simulink model "NL_RE"  (R2015a)
settings: Solver=ode4  StartTime=0.0  StopTime=10.0  RelTol=1e-3
values from neighbouring files (symbols this model uses):
  K = [0 K(2)]    [CommandeEE2.m]
undefined symbols (not defined in the file or in its folder): Cn, EE2, EE2_bf, J2, Kc, Ke, Kg, Kr, Ks, L, mu, obsver, R, Rchn, rCn, rRch
settings Model: Creator=sylvain  LastModifiedBy=Lucien
settings OptimizationCC: ExpressionDepthLimit=2147483647
settings DebuggingCC: UnderspecifiedInitializationDetection=Classic  MergeDetectMultiDrivingBlocksExec=none  SolverPrmCheckMsg=warning  StateNameClashWarn=warning

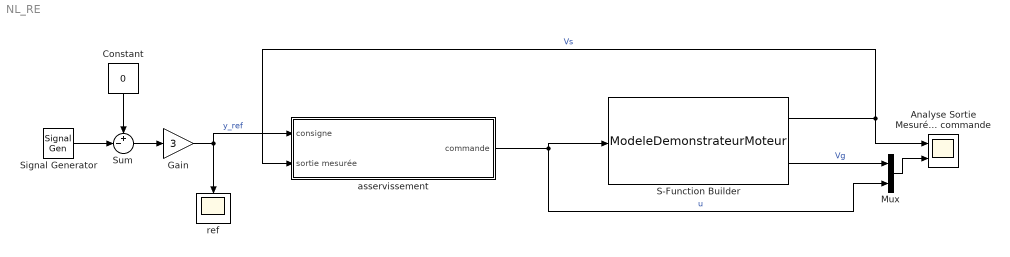
== system NL_RE ==
  Analyse Sortie Mesurée et commande : Scope  NumInputPorts=2
      settings: YMin=0.01~-5  YMax=0.0675~5
  Constant : Constant  Value=0
  Gain : Gain  Gain=3
  Mux : Mux  Inputs=2
  S-Function Builder : S-Function  InitFcn=try, set_param(gcb,'FunctionName','ModeleDemonstrateurMoteur'), end  FunctionName=ModeleDemonstrateurMoteur  Parameters=R,L,Ke,Kc,mu,J2,Cn,rCn,2*rand(1)-1,Ks,Kr,Kg,0.01,Rchn,rRch,2*rand(1)-1  SFunctionModules=ModeleDemonstrateurMoteur_wrapper  mask(S-Function Builder){}
      mask help: Simulink:masks:SFunctionBuilder_MD
      mask init:
      | val = [[.9  0.75 0.75 1 1 .9 .9 1]',[1 1 0.75 0.75 .9 .9 1 .9]'];try , sys = get_param(gcb,'SfunBuilderFcnName');if isempty(sys), sys = get_param(gcb,'FunctionName'); end,catch, sys = get_param(gcb,'FunctionName'); end
      settings: CopyFcn=set_param(gcbh,'LinkStatus','none')  PreSaveFcn=try, set_param(gcb,'FunctionName','ModeleDemonstrateurMoteur'), end  OpenFcn=sfunctionwizard(gcbh)
      mask Display: plot(val(:,1),val(:,2)),disp(sys), port_label('input',1,'Vm'), port_label('output',1,'Vs'), port_label('output',2,'Vg')
  Signal Generator : SignalGenerator  WaveForm=square  Frequency=0.2
  Sum : Sum  Inputs=+-|
  asservissement : Subsystem
  ref : Scope
      settings: SaveName=ScopeData3
  wires:
  Signal Generator/1 -> Sum/2
  Constant/1 -> Sum/1
  Sum/1 -> Gain/1
  Gain/1 -> asservissement/1(consigne), ref/1  "y_ref"
  Mux/1 -> Analyse Sortie Mesurée et commande/2
  S-Function Builder/1 -> asservissement/2(sortie mesurée), Analyse Sortie Mesurée et commande/1  "Vs"
  S-Function Builder/2 -> Mux/1  "Vg"
  asservissement/1(commande) -> S-Function Builder/1, Mux/2  "u"

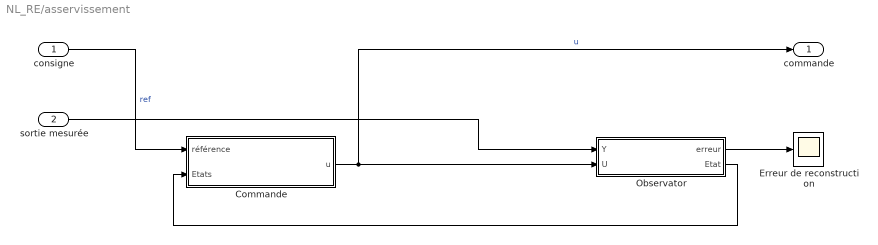
== system NL_RE/asservissement ==
  consigne : Inport
  sortie mesurée : Inport  Port=2
  "Commande " : Subsystem
  Erreur de reconstruction : Scope
      settings: SaveName=ScopeData4
  Observator : Subsystem
  commande : Outport
  wires:
  consigne/1 -> "Commande "/1(référence)  "ref"
  Observator/2("Etat ") -> "Commande "/2(Etats)
  sortie mesurée/1 -> Observator/1("Y ")
  "Commande "/1(u) -> Observator/2(U), commande/1  "u"
  Observator/1(erreur) -> Erreur de reconstruction/1

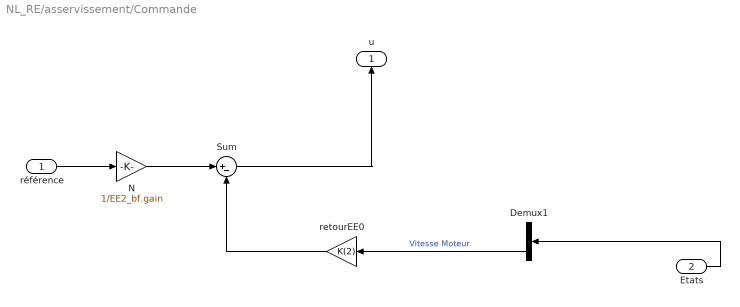
== system NL_RE/asservissement/Commande  ==
  référence : Inport
  Etats : Inport  Port=2
  Demux1 : Demux  Outputs=2
  "N " : Gain  Gain=1/EE2_bf.gain
  Sum : Sum  Inputs=|+-
  retourEE0 : Gain  Gain=K(2)
  u : Outport
  wires:
  Sum/1 -> u/1
  référence/1 -> "N "/1
  Etats/1 -> Demux1/1
  retourEE0/1 -> Sum/2
  "N "/1 -> Sum/1
  Demux1/2 -> retourEE0/1  "Vitesse Moteur"

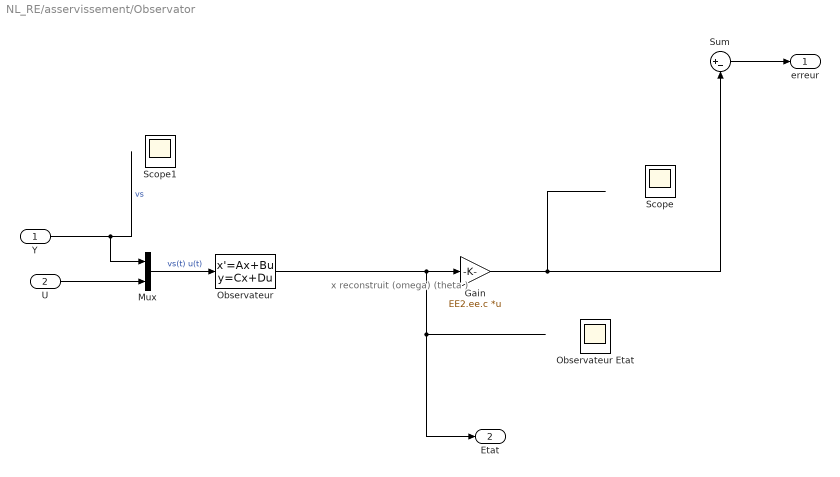
== system NL_RE/asservissement/Observator ==
  note: x reconstruit
      | (omega)
      | (theta   )
  "Y " : Inport
  U : Inport  Port=2
  Gain : Gain  Gain=EE2.ee.c  Multiplication=Matrix(K*u)
  Mux : Mux  Inputs=2
  "Observateur " : StateSpace  A=obsver.ee.a  B=obsver.ee.b  C=obsver.ee.c  D=obsver.ee.d  X0=0
  "Observateur Etat " : Scope
  Scope : Scope
      settings: YMin=-600  YMax=600
  Scope1 : Scope
      settings: YMin=16  YMax=30  SaveName=ScopeData2
  Sum : Sum  Inputs=|+-
  erreur : Outport
  "Etat " : Outport  Port=2
  wires:
  "Observateur "/1 -> "Etat "/1, Gain/1
  "Y "/1 -> Mux/1  "vs"
  Sum/1 -> erreur/1
  Mux/1 -> "Observateur "/1  "vs(t) u(t)"
  Gain/1 -> Sum/2
  U/1 -> Mux/2
